simulink model "fromWorkSpace_TestGen12"  (R2017b)
settings: Solver=FixedStepDiscrete  StartTime=0.0  StopTime=10.0  RelTol=1e-3
model workspace (MAT data in the model file):
  X_timeseries = timeseries
  X_timeseries.Name = 'unnamed'
  X_timeseries.DataInfo = tsdata.datametadata
  X_timeseries.DataInfo.Interpolation = tsdata.interpolation
  X_timeseries.DataInfo.Interpolation.Fhandle : function handle (value not decoded)
  X_timeseries.DataInfo.Interpolation.Name = 'linear'
  X_timeseries.TimeInfo = tsdata.timemetadata
  X_timeseries.TimeInfo.Length = 50
  X_timeseries.TimeInfo.DuplicateTimes = 0
  X_timeseries.TimeInfo.Time_ = [0; 0.2; 0.4; 0.6; 0.8; 1; 1.2; 1.4; 1.6; 1.8; 2; 2.2; 2.4; 2.6; 2.8; 3; 3.2; 3.4; 3.6; 3.8; 4; 4.2; 4.4; 4.6; 4.8; 5; 5.2; 5.4; 5.6; 5.8; 6; 6.2; 6.4; 6.6; 6.8; 7; 7.2; 7.4; 7.6; 7.8; 8; 8.2; 8.4; 8.6; 8.8; 9; 9.2; 9.4; 9.6; 9.8]
  X_timeseries.TimeInfo.Initialized = 1
  X_timeseries.QualityInfo = tsdata.qualmetadata
  X_timeseries.Data_ = [0.383644610643 0.158130466938 0.641884326935 0.038408331573 0.0668494328856 0.538985908031 0.918255269527 0.166713044047 0.124609671533 0.0136945899576 0.762762665749 0.722754180431 ... (1200 elements, 2x3x4x50)]
undefined symbols (not defined in the file): Block_TestLib, enable_trigger
settings Model: Creator=ktrinh  LastModifiedBy=ktrinh
settings DebuggingCC: ParameterOverflowMsg=none

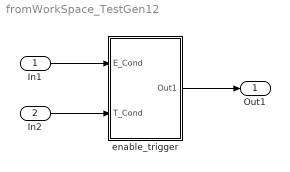
== system fromWorkSpace_TestGen12 ==
  In1 : Inport
  In2 : Inport  Port=2
  enable_trigger : Subsystem  AncestorBlock=Block_TestLib/enable_trigger
  Out1 : Outport
  wires:
  In1/1 -> enable_trigger/1(E_Cond)
  In2/1 -> enable_trigger/2(T_Cond)
  enable_trigger/1(Out1) -> Out1/1

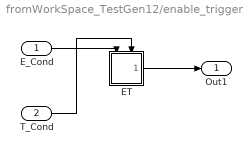
== system fromWorkSpace_TestGen12/enable_trigger ==
  E_Cond : Inport  OutDataTypeStr=boolean
  T_Cond : Inport  Port=2  OutDataTypeStr=boolean
  ET : Subsystem  TreatAsAtomicUnit=on
  Out1 : Outport
  wires:
  T_Cond/1 -> ET/Trigger
  E_Cond/1 -> ET/Enable
  ET/1(Out1) -> Out1/1

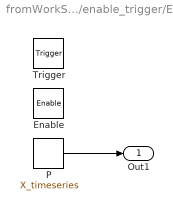
== system fromWorkSpace_TestGen12/enable_trigger/ET ==
  Enable : EnablePort
  Trigger : TriggerPort  VariantControl=Variant
  P : FromWorkspace  VariableName=X_timeseries  OutDataTypeStr=single  OutputAfterFinalValue=Holding final value
  Out1 : Outport
  wires:
  P/1 -> Out1/1
